simulink model "w2_prob3"  (R2020b)
settings: Solver=ode45  StartTime=0.0  StopTime=120  RelTol=1e-3
values from neighbouring files (symbols this model uses):
  b = 50    [w2_prob2matfile.m]
  m = 1000    [w2_prob2matfile.m]
settings Model: Creator=Akshay A H  LastModifiedBy=Akshay A H

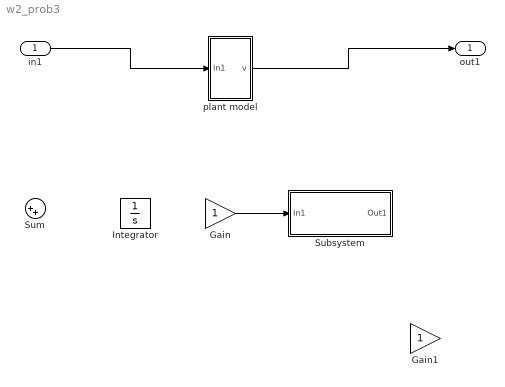
== system w2_prob3 ==
  in1 : Inport
  Gain : Gain
  Gain1 : Gain
  Integrator : Integrator
  Subsystem : Subsystem
  Sum : Sum  Inputs=|++
  plant model : Subsystem
  out1 : Outport
  wires:
  in1/1 -> plant model/1(In1)
  plant model/1(v) -> out1/1
  Gain/1 -> Subsystem/1(In1)

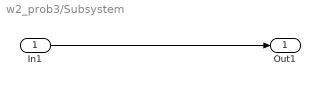
== system w2_prob3/Subsystem ==
  In1 : Inport
  Out1 : Outport
  wires:
  In1/1 -> Out1/1

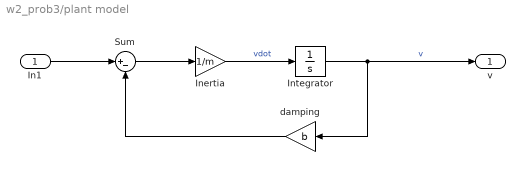
== system w2_prob3/plant model ==
  In1 : Inport
  Inertia : Gain  Gain=1/m
  Integrator : Integrator
  Sum : Sum  Inputs=|+-
  damping : Gain  Gain=b
  v : Outport
  wires:
  Inertia/1 -> Integrator/1  "vdot"
  Sum/1 -> Inertia/1
  In1/1 -> Sum/1
  damping/1 -> Sum/2
  Integrator/1 -> v/1, damping/1  "v"
